simulink model "closed_loop_model_3_1"  (R2023b)
settings: Solver=ode1  StartTime=0.0  StopTime=30  FixedStep=0.001  RelTol=1e-3
values from neighbouring files (symbols this model uses):
  d = 0.4    [problem_3_1.m]
  k = 2200    [problem_3_1.m]
  m1 = 0.015    [problem_3_1.m]
  m2 = 0.0045    [problem_3_1.m]
settings Model: Creator=sarth  LastModifiedBy=sarth

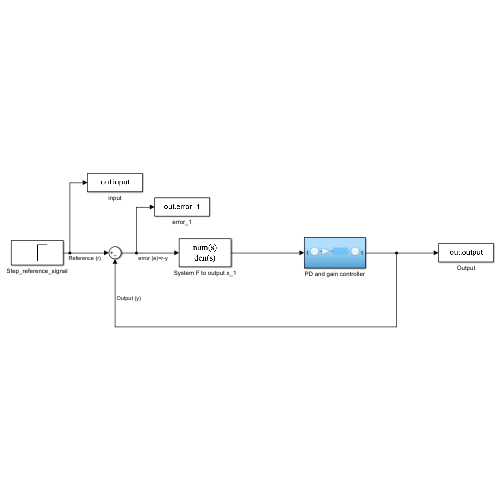
[thumbnail: Simulink's stored preview of the top-level diagram]
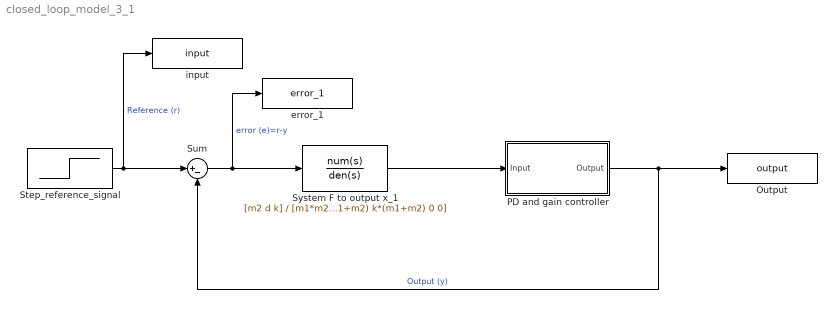
== system closed_loop_model_3_1 ==
  Output : ToWorkspace  VariableName=output  SampleTime=-1
  PD and gain controller : Subsystem
  Step_reference_signal : Step  SampleTime=0.001
  Sum : Sum  Inputs=|+-
  System F to output x_1 : TransferFcn  Numerator=[m2 d k]  Denominator=[m1*m2 d*(m1+m2) k*(m1+m2) 0 0]
  error_1 : ToWorkspace  VariableName=error_1  SampleTime=-1
  input : ToWorkspace  VariableName=input  SaveFormat=Timeseries  SampleTime=-1
  wires:
  System F to output x_1/1 -> PD and gain controller/1(Input)
  Sum/1 -> error_1/1, System F to output x_1/1  "error (e)=r-y"
  Step_reference_signal/1 -> input/1, Sum/1  "Reference (r)"
  PD and gain controller/1(Output) -> Sum/2, Output/1  "Output (y)"

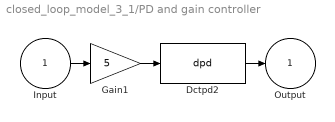
== system closed_loop_model_3_1/PD and gain controller ==
  Input : Inport
  Dctpd2 : S-Function  FunctionName=dpd  Parameters=kp, kv, 0.001  SFunctionDeploymentMode=off  EnableBusSupport=off  mask(dctools){kp=36.5, kv=0.4}
      mask help: This block implements a discrete time pd filter.
      mask Display: disp('DCT pd')
  Gain1 : Gain  Gain=5
  Output : Outport
  wires:
  Input/1 -> Gain1/1
  Gain1/1 -> Dctpd2/1
  Dctpd2/1 -> Output/1
